simulink model "stage13"  (Simulink 7.7)
settings: Solver=ode45  StartTime=0.0  StopTime=10  RelTol=1e-3
undefined symbols (not defined in the file): Acid, Capacitor, Lead, Run, Start
libraries: powerlib x20, simulink x4, fl_lib x4, powerlib_extras x3, nesl_utility x3, electricdrivelib x2, elec_lib x2
settings Model: Creator=Vikas  LastModifiedBy=Vikas

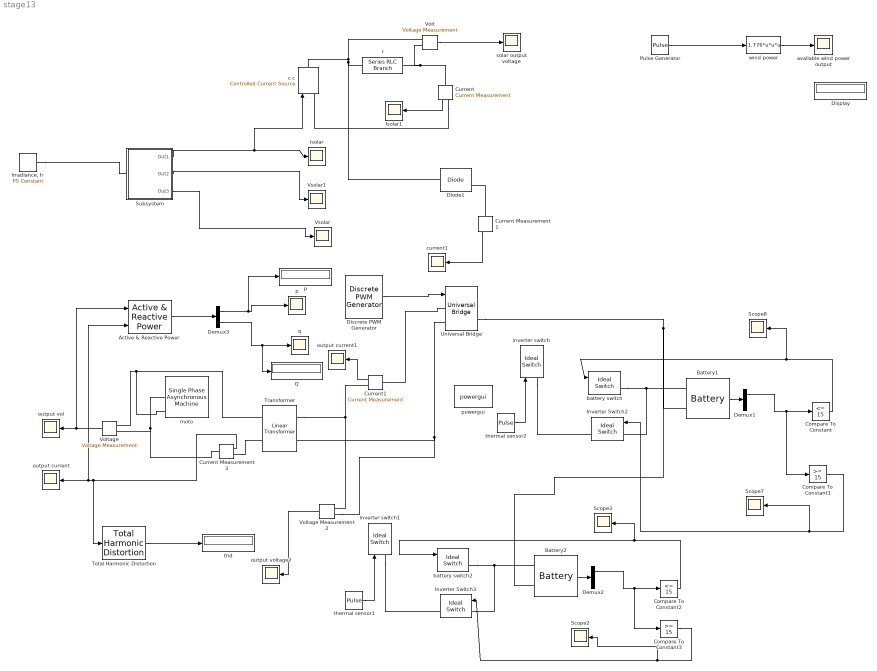
== system stage13 ==
  Active & Reactive Power : powerlib_extras/Measurements/Active & Reactive Power  SystemSampleTime=-1  f1=50
  Battery1 : electricdrivelib/Extra Sources/Battery  SystemSampleTime=-1  BatType=Lead-Acid  ShowDetailedParameters=off  NomV=15  NomQ=60  SOC=0  PresetModel=on  MaxQ=62.5  FullV=16.3322  Dis_rate=12  R=0.0025  Normal_OP=18.6167  expZone="[15.2714          0.2]"  Dis_Char=off  current=[6.5 13 32.5]  Units=Time  Batt_Tr=5
  Battery2 : electricdrivelib/Extra Sources/Battery  SystemSampleTime=-1  BatType=Lead-Acid  ShowDetailedParameters=off  NomV=15  NomQ=60  SOC=100  PresetModel=on  MaxQ=62.5  FullV=16.3322  Dis_rate=12  R=0.0025  Normal_OP=18.6167  expZone="[15.2714          0.2]"  Dis_Char=off  current=[6.5 13 32.5]  Units=Time  Batt_Tr=5
  Compare To Constant : simulink/Logic and Bit Operations/Compare To Constant  SystemSampleTime=-1  relop=<=  const=15  LogicOutDataTypeMode=uint8
  Compare To Constant1 : simulink/Logic and Bit Operations/Compare To Constant  SystemSampleTime=-1  relop=>=  const=15  LogicOutDataTypeMode=uint8
  Compare To Constant2 : simulink/Logic and Bit Operations/Compare To Constant  SystemSampleTime=-1  relop=<=  const=15  LogicOutDataTypeMode=uint8
  Compare To Constant3 : simulink/Logic and Bit Operations/Compare To Constant  SystemSampleTime=-1  relop=>=  const=15  LogicOutDataTypeMode=uint8
  Current : powerlib/Measurements/Current Measurement  SystemSampleTime=-1  PhasorSimulation=off  OutputType=Complex  PSBequivalent=0
  Current Measurement1 : powerlib/Measurements/Current Measurement  SystemSampleTime=-1  PhasorSimulation=off  OutputType=Complex  PSBequivalent=0
  Current Measurement3 : powerlib/Measurements/Current Measurement  SystemSampleTime=-1  PhasorSimulation=off  OutputType=Complex  PSBequivalent=0
  Current1 : powerlib/Measurements/Current Measurement  SystemSampleTime=-1  PhasorSimulation=off  OutputType=Complex  PSBequivalent=0
  Demux1 : Demux  Outputs=3
  Demux2 : Demux  Outputs=3
  Demux3 : Demux  Outputs=2
  Diode1 : powerlib/Power Electronics/Diode  SystemSampleTime=-1  Ron=0.001  Lon=0  Vf=0.8  IC=0  UseSnubber=off  Rs=500  Cs=250e-9  Measurements=on
  Discrete PWM Generator : powerlib_extras/Discrete  Control Blocks/Discrete PWM Generator  SystemSampleTime=-1  GeneratorMode="2-arm  bridge (4 pulses)"  Fc=5000  Ts=5e-6  Internal=on  mIndex=0.4  Freq=50  Phase=0
  Display : Display
  Inverter Switch2 : powerlib/Power Electronics/Ideal Switch  SystemSampleTime=-1  Ron=0.001  Lon=0  IC=0  Rs=1e5  Cs=inf  Measurements=on
  Inverter Switch3 : powerlib/Power Electronics/Ideal Switch  SystemSampleTime=-1  Ron=0.001  Lon=0  IC=0  Rs=1e5  Cs=inf  Measurements=on
  "Irradiance, Ir" : fl_lib/Physical Signals/Sources/PS Constant  SystemSampleTime=-1  constant=1000  LocalVarLogging=[]
  Isolar : Scope
      settings: TimeRange=1  YMin=2  YMax=8  SaveName=Io
  Isolar1 : Scope
      settings: TimeRange=1  YMin=2.23577  YMax=2.23577  SaveName=Io1
  P : Display
  Pulse Generator : DiscretePulseGenerator  PulseType=Time based  Amplitude=3.84  Period=10  PulseWidth=50
  Q : Display
  Scope{2..3,7..8} (4 alike) : Scope
      Scope2 settings: TimeRange=0.1  YMin=0.95  YMax=1.05  SaveName=ScopeData5
      Scope3 settings: TimeRange=0.02  YMin=0.95  YMax=1.05  SaveName=ScopeData10
      Scope7 settings: TimeRange=0.1  YMin=0.95  YMax=1.05  SaveName=ScopeData7
      Scope8 settings: TimeRange=0.02  YMin=0.95  YMax=1.05  SaveName=ScopeData9
  Subsystem : Subsystem
  Total Harmonic Distortion : powerlib_extras/Measurements/Total Harmonic Distortion  SystemSampleTime=-1  f1=50
  Transformer : powerlib/Elements/Linear Transformer  PhysicalDomain=powersysdomain  SubClassName=unknown  LeftPortType=p1  RightPortType=p1  LConnTagsString=a|b  RConnTagsString=A|B  UNITS=pu  NominalPower=[ 875 50 ]  winding1=[12 0.002 0]  winding2=[240 0.002 0.0]  ThreeWindings=off  winding3=[3.15e+005 0.002 0.08]  RmLm=[500 500]  Measurements=None  DataType=off
  Universal Bridge : powerlib/Power Electronics/Universal Bridge  SystemSampleTime=-1  Arms=2  SnubberResistance=1e5  SnubberCapacitance=inf  Device=MOSFET / Diodes  Ron=1e-3  Lon=0  ForwardVoltages="[  0  0  ]"  ForwardVoltage=0  GTOparameters=[ 10e-6 , 20e-6 ]  IGBTparameters=[ 1e-6 , 2e-6 ]  Measurements=None  Measurements_2=None  converterType=Rectifier
  Volt : powerlib/Measurements/Voltage Measurement  SystemSampleTime=-1  PhasorSimulation=off  OutputType=Complex  PSBequivalent=0
  Voltage : powerlib/Measurements/Voltage Measurement  SystemSampleTime=-1  PhasorSimulation=off  OutputType=Complex  PSBequivalent=0
  Voltage Measurement2 : powerlib/Measurements/Voltage Measurement  SystemSampleTime=-1  PhasorSimulation=off  OutputType=Complex  PSBequivalent=0
  Vsolar : Scope
      settings: TimeRange=1  YMin=0  YMax=0.8  SaveName=Vo
  Vsolar1 : Scope
      settings: TimeRange=1  YMin=0  YMax=0.8  SaveName=Vo1
  available wind power output : Scope
      settings: TimeRange=0.1  YMin=265.673  YMax=293.639  SaveName=ScopeData13
  battery switch : powerlib/Power Electronics/Ideal Switch  SystemSampleTime=-1  Ron=0.001  Lon=0  IC=0  Rs=1e5  Cs=inf  Measurements=on
  battery switch2 : powerlib/Power Electronics/Ideal Switch  SystemSampleTime=-1  Ron=0.001  Lon=0  IC=0  Rs=1e5  Cs=inf  Measurements=on
  c c : powerlib/Electrical Sources/Controlled Current Source  SystemSampleTime=-1  Initialize=on  Source_Type=DC  Amplitude=1  Phase=0  Frequency=0  Measurements=None
  current1 : Scope
      settings: TimeRange=0.04  YMin=2.11441  YMax=2.11442  SaveName=ScopeData11
  inverter switch : powerlib/Power Electronics/Ideal Switch  SystemSampleTime=-1  Ron=0.001  Lon=0  IC=0  Rs=1e5  Cs=inf  Measurements=on
  inverter switch1 : powerlib/Power Electronics/Ideal Switch  SystemSampleTime=-1  Ron=0.001  Lon=0  IC=0  Rs=1e5  Cs=inf  Measurements=on
  moto : powerlib/Machines/Single Phase Asynchronous Machine  SystemSampleTime=-1  UNITS=SI  MachineType=Capacitor-Start-Run  NominalParameters="[ 133.33  230  50]"  MainWindingStator="[2.02  7.4e-3]"  MainWindingRotor="[4.12  5.6e-3]"  MutualInductance=0.1772  AuxiliaryWinding="[7.14  8.5e-3]"  Mechanical="[0.0146  0  2 1.18]"  CapacitorStart="[2  254.7e-6]"  CapacitorRun="[18  21.1e-6]"  DisconnectionSpeed=75  InitialSpeed=0  DataType=SI  TsPowergui=0  TsBlock=-1
  output current : Scope
      settings: TimeRange=0.1  YMin=-50  YMax=50  SaveName=ScopeData15
  output current1 : Scope
      settings: TimeRange=0.1  YMin=-50  YMax=50  SaveName=ScopeData16
  output vol : Scope
      settings: YMin=-375  YMax=25  SaveName=ScopeData12
  output voltage2 : Scope
      settings: YMin=-17.5  YMax=17.5  SaveName=ScopeData8
  p : Scope
      settings: TimeRange=1  YMin=846  YMax=862  SaveName=Vo4
  powergui : powerlib/powergui  Priority=1  SystemSampleTime=-1  SimulationMode=Discrete  SampleTime=1e-6  frequency=60  SPID=off  DisableSnubberDevices=off  DisableRonSwitches=off  DisableVfSwitches=off  SwTol=0  Interpol=off  DisplayEquations=off  FunctionMessages=off  frequencyindice=0  Pbase=100e6  ErrMax=1e-4  Iterations=50  UnitsV=kV  UnitsW=MW  echomessages=off  HookPort=off  EnableUseOfTLC=off  x0status=steady  RestoreLinks=no  ResistiveCurrentMeasurement=off  Frange=[0:2:500]  Ylog=off  Xlog=on  ShowGrid=off  save=off  variable=ZData  structure=ScopeData8  ZoomFFT=off  StartTime=0.0  cycles=1  DisplayStyle=1  fundamental=60  FreqAxis=off  MaxFrequency=1000  frequencyindicesteady=1  RmsSteady=1  display=off  Ts=0  methode=off
  q : Scope
      settings: TimeRange=1  YMin=0  YMax=0.8  SaveName=Vo5
  r : powerlib/Elements/Series RLC Branch  PhysicalDomain=powersysdomain  SubClassName=unknown  LeftPortType=p1  RightPortType=p1  LConnTagsString=__new0  RConnTagsString=__new0  BranchType=R  Resistance=6.75  Inductance=1e-3  SetiL0=off  InitialCurrent=0  Capacitance=1e-6  Setx0=off  InitialVoltage=0  Measurements=None
  solar output voltage : Scope
      settings: YMin=0  SaveName=ScopeData14
  thd : Display
  thermal sensor1 : DiscretePulseGenerator  PulseType=Time based  Period=14400  PulseWidth=50
  thermal sensor2 : DiscretePulseGenerator  PulseType=Time based  Period=14400  PulseWidth=50
  "wind power " : Fcn  Expr=1.776*u*u*u
  wires:
  Battery1/1 -> Demux1/1
  Demux1/1 -> Compare To Constant/1, Compare To Constant1/1
  Compare To Constant/1 -> Scope8/1, battery switch/1
  Compare To Constant1/1 -> Inverter Switch2/1, Scope7/1
  thermal sensor2/1 -> inverter switch/1
  Pulse Generator/1 -> "wind power "/1
  "wind power "/1 -> available wind power output/1
  Voltage/1 -> output vol/1, Active & Reactive Power/1
  Voltage Measurement2/1 -> output voltage2/1
  Discrete PWM Generator/1 -> Universal Bridge/1
  Battery2/1 -> Demux2/1
  Demux2/1 -> Compare To Constant2/1, Compare To Constant3/1
  Compare To Constant2/1 -> battery switch2/1, Scope3/1
  Compare To Constant3/1 -> Inverter Switch3/1, Scope2/1
  thermal sensor1/1 -> inverter switch1/1
  Subsystem/2(Out2) -> Vsolar1/1
  Current/1 -> Isolar1/1
  Volt/1 -> solar output voltage/1
  Current Measurement3/1 -> output current/1, Active & Reactive Power/2, Total Harmonic Distortion/1
  Current Measurement1/1 -> current1/1
  Active & Reactive Power/1 -> Demux3/1
  Demux3/1 -> p/1, P/1
  Demux3/2 -> q/1, Q/1
  Subsystem/1(Out1) -> Isolar/1, c c/1
  Subsystem/3(Out3) -> Vsolar/1
  Total Harmonic Distortion/1 -> thd/1
  Current1/1 -> output current1/1
  connections:
  Battery1/LConn1 -- battery switch/RConn1 -- Inverter Switch2/LConn1
  inverter switch/LConn1 -- Inverter Switch2/RConn1
  moto/LConn2 -- Transformer/RConn1 -- Voltage/LConn1
  Voltage Measurement2/LConn2 -- Universal Bridge/LConn2 -- Transformer/LConn2
  Inverter Switch3/LConn1 -- Battery2/LConn1 -- battery switch2/RConn1
  inverter switch1/LConn1 -- Inverter Switch3/RConn1
  Universal Bridge/RConn2 -- Battery2/LConn2 -- Battery1/LConn2
  r/RConn1 -- Volt/LConn1 -- c c/RConn1 -- Diode1/LConn1
  Current/RConn1 -- c c/LConn1
  "Irradiance, Ir"/RConn1 -- Subsystem/LConn1
  Current Measurement3/LConn1 -- moto/LConn1 -- Voltage/LConn2
  Current Measurement1/LConn1 -- Diode1/RConn1
  Current Measurement3/RConn1 -- Transformer/RConn2
  Transformer/LConn1 -- Voltage Measurement2/LConn1 -- Current1/RConn1
  Universal Bridge/LConn1 -- Current1/LConn1
  Volt/LConn2 -- r/LConn1 -- Current/LConn1

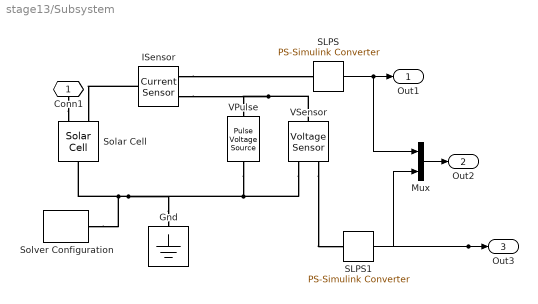
== system stage13/Subsystem ==
  Gnd : fl_lib/Electrical/Electrical Elements/Electrical Reference  SystemSampleTime=-1  i_Log=off  LocalVarNames=|i  LocalVarDescs=|i  LocalVarLogging=[]
  ISensor : fl_lib/Electrical/Electrical Sensors/Current Sensor  SystemSampleTime=-1  i1_Log=off  v1_Log=off  LocalVarNames=|i1|v1  LocalVarDescs=|i1|v1  LocalVarLogging=[0 0]
  Mux : Mux  Inputs=2
  SLPS : nesl_utility/PS-Simulink Converter  SystemSampleTime=-1  PhysicalDomain=network_engine_domain  LeftPortType=input  RightPortType=output  SubClassName=ps_output  Unit=A  AffineConversion=off
  SLPS1 : nesl_utility/PS-Simulink Converter  SystemSampleTime=-1  PhysicalDomain=network_engine_domain  LeftPortType=input  RightPortType=output  SubClassName=ps_output  Unit=V  AffineConversion=off
  Solar Cell : elec_lib/Sources/Solar Cell  SystemSampleTime=-1  prm=1  Isc=7.34 A  Voc=0.6 V  Is=1e-06 A  Is2=0 A  Iph=7.34 A  Ir0=1000 W/m^2  ec=1.5  N2=2  Rs=0 Ohm  Rp=Inf Ohm  TIPH1=0 1/K  EG=1.11 eV  TXIS1=3  TXIS2=3  TRS1=0  TRP1=0  TFIXED=25 C  Tmeas=25 C  LocalVarLogging=[]
  Solver Configuration : nesl_utility/Solver Configuration  SystemSampleTime=-1  PhysicalDomain=network_engine_domain  LeftPortType=input  RightPortType=generic  SubClassName=solver  Accelerate=off  Profile=off  ResidualTolerance=1e-9  MaxNonlinIter=3  MaxModeIter=2  DoFixedCost=off  UseLocalSampling=off  DoDC=off  LinearAlgebra=Sparse  LocalSolverSampleTime=.001  LocalSolverChoice=NE_BACKWARD_EULER_ADVANCER  UseLocalSolver=off
  VPulse : elec_lib/Additional Components/SPICE-Compatible Components/Sources/Pulse Voltage Source  SystemSampleTime=-1  V1=0 V  V2=0 V  TD=0 s  TR=1 s  TF=0 s  PW=Inf s  PER=Inf s  voltage_Log=off  LocalVarNames=|voltage  LocalVarDescs=|Voltage (V)  LocalVarLogging=0
  VSensor : fl_lib/Electrical/Electrical Sensors/Voltage Sensor  SystemSampleTime=-1  i1_Log=off  v1_Log=off  LocalVarNames=|i1|v1  LocalVarDescs=|i1|v1  LocalVarLogging=[0 0]
  Conn1 : PMIOPort  Port=1  Side=Left
  Out1 : Outport
  Out2 : Outport  Port=2
  Out3 : Outport  Port=3
  wires:
  SLPS1/1 -> Mux/2, Out3/1
  SLPS/1 -> Mux/1, Out1/1
  Mux/1 -> Out2/1
  connections:
  Gnd/LConn1 -- Solar Cell/RConn1 -- Solver Configuration/RConn1 -- VPulse/RConn1 -- VSensor/RConn2
  ISensor/LConn1 -- Solar Cell/LConn2
  ISensor/RConn1 -- SLPS/LConn1
  ISensor/RConn2 -- VPulse/LConn1 -- VSensor/LConn1
  VSensor/RConn1 -- SLPS1/LConn1
  Conn1/RConn1 -- Solar Cell/LConn1
